simulink model "pos_control2"  (R2016b)
settings: Solver=ode3  StartTime=0.0  StopTime=50  FixedStep=0.0025  RelTol=1e-3
model workspace: external: MATLAB File /home/zhouhua/Clobotics/px4_simulink/px4_motor_order/pos_control_px4_order/para_pos.m (data not in the file)
values from neighbouring files (symbols this model uses):
  Ang_Pos_initial = [x0, y0, z0, phi0, theta0, psi0]    [para_pos.m]
  b = (middle_cruise_speed - c) / a    [get_vel_close.m]    (also in gradual.m = y_low - a * x_low; para_pos.m = 1.38089806e-06)
  compensation_gain = 1    [para_pos.m]
  d = 4.152245751114358e-08    (= 4.15224575111e-08)    [para_pos.m]
  dt = 0.0025    [para_pos.m]
  g = 9.8    [para_pos.m]
  Ix = 0.676603    [para_pos.m]
  Iy = 0.996394    [para_pos.m]
  Iz = 0.640393    [para_pos.m]
  L = 0.6    [para_pos.m]
  m = 10.3551    [para_pos.m]
  omiga1 = 0000    (= 0)    [para_pos.m]
  omiga2 = 0000    (= 0)    [para_pos.m]
  omiga3 = 0000    (= 0)    [para_pos.m]
  omiga4 = 0000    (= 0)    [para_pos.m]
  thrust_rpyt_low = [0,0,0,0,0,0]    [para_pos.m]
  thrust_rpyt_up = [1,1,1,1,1,1]    [para_pos.m]
  X1_PWM_MotorVel = -0.0023    [para_pos.m]
  X2_PWM_MotorVel = 13.6492    [para_pos.m]
  X3_PWM_MotorVel = -1.2185e+4    (= -12185)    [para_pos.m]
undefined symbols (not defined in the file or in its folder): bool_pos, control_mode, def, par, par_input, par_pos, position_setpoint
libraries: simulink x1
(part 2 of 2)

== matlab function pos_control2/position_control/control_auto ==
  data: prev_pos_sp input; next_sp input; curr_pos_sp input; pos input; vel input; att_euler input; vel_sp_prev input; pos_sp_prev input; att_sp_prev_yaw_body input; pos_sp_x output; pos_sp_y output; pos_sp_z output; vel_sp_x output; vel_sp_y output; vel_sp_z output; att_sp_yaw_body output; vel_max_xy output; def parameter; bool_pos parameter; position_setpoint parameter; par_pos parameter; dt parameter
function [pos_sp_x,pos_sp_y,pos_sp_z,vel_sp_x,vel_sp_y,vel_sp_z,att_sp_yaw_body,vel_max_xy] = control_auto(prev_pos_sp,next_sp,curr_pos_sp,pos,vel,att_euler,vel_sp_prev,pos_sp_prev,att_sp_prev_yaw_body,def, bool_pos, position_setpoint,par_pos, dt)
%curr_pos_sp(valid,type,x,y,z,vx,vy,vz,ax,ay,az,yaw,yawspeed,cruising_speed,position_valid,velocity_valid,acceleration_valid,yaw_valid,yawspeed_valid,cruising_valid)
%[1,0,10,10,10,0.1,0.1,0.1,0,0,0,1,0.1,0,1,1,0,1,0,0]
%prev_sp,next_sp [valid,type,x,y,z]
vel_max_xy = par_pos.vel_max_xy;
pos_sp = zeros(3,1);
pos_sp = pos_sp_prev;
vel_sp = zeros(3,1);
vel_sp = vel_sp_prev;
yaw = att_euler(3);
att_sp_yaw_body = att_sp_prev_yaw_body;
% reset position setpoint on AUTO mode activation or if we are not in MC mode */
if ~bool_pos.mode_auto
    bool_pos.mode_auto = 1;
    %set _triplet_lat_lon_finite true once switch to AUTO(e.g. LAND)
    bool_pos.triplet_lat_lon_finite = 1;

end

bool_pos.reset_pos_sp = 1;
bool_pos.reset_alt_sp = 1;

% Always check reset state of altitude and position control flags in auto
if (bool_pos.reset_pos_sp)
   bool_pos.reset_pos_sp = 0;
   pos_sp(1) = pos(1);
   pos_sp(2) = pos(2);
end

if (bool_pos.reset_alt_sp)
    bool_pos.reset_alt_sp = 0;
    pos_sp(3) = pos(3);
end

% init bool and vector
%bool
current_setpoint_valid = 0;
previous_setpoint_valid = 0;
next_setpoint_valid = 0;
triplet_updated = 0;

if (curr_pos_sp(1))

    %math::Vector<3> 
    %curr_pos_sp = _curr_pos_sp;

    %only project setpoints if they are finite, else use current position
     
    %if (PX4_ISFINITE(_pos_sp_triplet.current.lat) &&
       % PX4_ISFINITE(_pos_sp_triplet.current.lon)) {
        % project setpoint to local frame */
        %map_projection_project(&_ref_pos, _pos_sp_triplet.current.lat, _pos_sp_triplet.current.lon,&curr_pos_sp.data[0], &curr_pos_sp.data[1]);

        %_triplet_lat_lon_finite = true;

    %} else { % use current position if NAN -> e.g. land
       % if (_triplet_lat_lon_finite) {
        %    curr_pos_sp.data[0] = _pos(0);
         %   curr_pos_sp.data[1] = _pos(1);
       %     _triplet_lat_lon_finite = false;
        %}
    % only project setpoints if they are finite, else use current position
    % todo ref_alt
    %if (PX4_ISFINITE(_pos_sp_triplet.current.alt)) {
        %curr_pos_sp(5) = -(_pos_sp_triplet.current.alt - _ref_alt);
   % }
    % sanity check */
    if (isreal(curr_pos_sp(3)) && isreal(curr_pos_sp(4)) && isreal(curr_pos_sp(5)))
        current_setpoint_valid = 1;
    end

    % check if triplets have been updated
    % note: we only can look at xy since navigator applies slewrate to z */
    %float  diff;
    %if (_triplet_lat_lon_finite) {
       % diff = matrix::Vector2f((_curr_pos_sp(0) - curr_pos_sp(0)), (_curr_pos_sp(1) - curr_pos_sp(1))).length();
    %} else {
       % diff = fabsf(_curr_pos_sp(2) - curr_pos_sp(2));
    %}
    %if (diff > FLT_EPSILON) {
    %    triplet_updated = true;
    %}
    % we need to update _curr_pos_sp always since navigator applies slew rate on z */
    %_curr_pos_sp = curr_pos_sp;
end

if (prev_pos_sp(1))
    if (isreal(prev_pos_sp(3)) && isreal(prev_pos_sp(4)) && isreal(prev_pos_sp(5)))
        %_prev_pos_sp = prev_sp;
        previous_setpoint_valid = 1;
    end
end

% set previous setpoint to current position if no previous setpoint available */
if (~previous_setpoint_valid && triplet_updated)
    prev_pos_sp(3) = pos(1);
    prev_pos_sp(4) = pos(2);
    prev_pos_sp(5) = pos(3);
    previous_setpoint_valid = 1; % currrently not necessary to set to true since not used*/
end

if (next_sp(1))
    if (isreal(next_sp(3)) && isreal(next_sp(4)) && isreal(next_sp(5)))
        next_setpoint_valid = 1;
    end
end

%change curr_pos_sp, prev_pos_sp, next_sp
%todo
%current_setpoint_valid = 1;

%create new _pos_sp from triplets
if (current_setpoint_valid && curr_pos_sp(2) ~= position_setpoint.SETPOINT_TYPE_IDLE)
    % update yaw setpoint if needed
    if (curr_pos_sp(19) && position_setpoint.SETPOINT_TYPE_FOLLOW_TARGET)
        att_sp_yaw_body = att_sp_prev_yaw_body + curr_pos_sp(13)*dt;
    elseif (curr_pos_sp(18))
        att_sp_yaw_body = curr_pos_sp(12);
    end
    
    yaw_diff = wrap_pi(att_sp_yaw_body - yaw);
    
    % only follow previous-current-line for specific triplet type
    
    if  (curr_pos_sp(2) == position_setpoint.SETPOINT_TYPE_POSITION  ||curr_pos_sp(2) == position_setpoint.SETPOINT_TYPE_LOITER ||curr_pos_sp(2) == position_setpoint.SETPOINT_TYPE_FOLLOW_TARGET)
        %by default use current setpoint as is
        pos_sp = [curr_pos_sp(3);curr_pos_sp(4);curr_pos_sp(5)];
        
        %Z-DIRECTION
        
        % get various distances
        
		total_dist_z = abs(curr_pos_sp(5) - prev_pos_sp(5));
		dist_to_prev_z = abs(pos(3) - prev_pos_sp(5));
		dist_to_current_z = abs(curr_pos_sp(5) - pos(3));
        
        %  if pos_sp has not reached target setpoint (=curr_pos_sp(2)),
		%  then compute setpoint depending on vel_max
        if (total_dist_z >  def.SIGMA_NORM) && (abs(pos_sp(3) - curr_pos_sp(5)) > def.SIGMA_NORM)
            %%% ???
            flying_upward = (curr_pos_sp(5) < pos(3));
            
            % final_vel_z is the max velocity which depends on the distance of total_dist_z
			% with default params.vel_max_up/down
            if flying_upward
                final_vel_z = par_pos.vel_max_up;
            else
                final_vel_z = par_pos.vel_max_down;
            end
            % target threshold defines the distance to _curr_pos_sp(2) at which
			% the vehicle starts to slow down to approach the target smoothly
            target_threshold_z = final_vel_z * 1.5;
            % if the total distance in z is NOT 2x distance of target_threshold, we
			% will need to adjust the final_vel_z
			is_2_target_threshold_z = total_dist_z >= 2.0 * target_threshold_z;
			
            slope = (final_vel_z) / (target_threshold_z); % defines the the acceleration when slowing down */
			min_vel_z = 0.2; % minimum velocity: this is needed since estimation is not perfect
            
            if (~is_2_target_threshold_z)
				% adjust final_vel_z since we are already very close
				% to current and therefore it is not necessary to accelerate
				% up to full speed (=final_vel_z)
				target_threshold_z = total_dist_z * 0.5;
				%get the velocity at target_threshold_z */
				final_vel_z_tmp = slope * (target_threshold_z) + min_vel_z;

				%make sure that final_vel_z is never smaller than 0.5 of the default final_vel_z
				%this is mainly done because the estimation in z is not perfect and therefore
				%it is necessary to have a minimum speed

				final_vel_z = constrain(final_vel_z_tmp, final_vel_z * 0.5, final_vel_z);
            end

			vel_sp_z = final_vel_z;

			%we want to slow down */
            if (dist_to_current_z < target_threshold_z) 
                vel_sp_z = slope * dist_to_current_z + min_vel_z;
            elseif (dist_to_prev_z < target_threshold_z)
				%we want to accelerate */

				acc_z = (vel_sp_z - abs(vel_sp(3))) / dt;
                if flying_upward
                    acc_max = par_pos.acceleration_z_max_up * 0.5;
                else
                    acc_max = par_pos.acceleration_z_max_down * 0.5;
                end
                
                if (acc_z > acc_max)
                    vel_sp_z = par_pos.acceleration_z_max_up * dt + abs(vel_sp(3));
                end

            end

			%if we already close to current, then just take over the velocity that
			%we would have computed if going directly to the current setpoint
            if (vel_sp_z >= (dist_to_current_z * par_pos.pos_p(3)))
				vel_sp_z = dist_to_current_z * par_pos.pos_p(3);
            end

			% make sure vel_sp_z is always positive */
			vel_sp_z = constrain(vel_sp_z, 0.0, final_vel_z);
			% get the sign of vel_sp_z */
            if flying_upward
                vel_sp_z = -vel_sp_z ;
            %else
               % vel_sp_z = vel_sp_z;
            end
			% compute pos_sp(2) */
			pos_sp(3) = pos(3) + vel_sp_z / par_pos.pos_p(3);
        end
        
        
        % XY-DIRECTION


		% line from previous to current and from pos to current */
        vec_prev_to_current = [(curr_pos_sp(3) - prev_pos_sp(3)); (curr_pos_sp(4) - prev_pos_sp(4))];
        vec_pos_to_current = [(curr_pos_sp(3) - pos(1)); (curr_pos_sp(4) - pos(2))];


		% check if we just want to stay at current position */
		pos_sp_diff = [(curr_pos_sp(3) - pos_sp(1)); (curr_pos_sp(4) - pos_sp(2))];
		% bool
        stay_at_current_pos = (curr_pos_sp(2) == position_setpoint.SETPOINT_TYPE_LOITER || ~next_setpoint_valid) && (normest(pos_sp_diff) < def.SIGMA_NORM);

        % only follow line if previous to current has a minimum distance */

		% only follow line if previous to current has a minimum distance */
        if ((normest(vec_prev_to_current)  > par_pos.nav_rad ) && ~stay_at_current_pos) 

			% normalize prev-current line (always > nav_rad) */
			unit_prev_to_current = vec_prev_to_current/normest(vec_prev_to_current);

			% unit vector from current to next */
			unit_current_to_next = [0.0; 0.0];
            
            if (next_setpoint_valid) 
					unit_current_to_next = [(next_sp(3) - pos_sp(1)); (next_sp(4) - pos_sp(2))];
                    if normest(unit_current_to_next) > def.SIGMA_NORM
                        unit_current_to_next = unit_current_to_next/normest(unit_current_to_next);
                    %else
                        %unit_current_to_next;
                    end
            end

			% point on line closest to pos */
			closest_point = [prev_pos_sp(3); prev_pos_sp(4)] + unit_prev_to_current * ([(pos(1) - prev_pos_sp(3)), (pos(2) - prev_pos_sp(4))] * unit_prev_to_current);

			vec_closest_to_current = [(curr_pos_sp(3) - closest_point(1)); (curr_pos_sp(4) - closest_point(2))];

			% compute vector from position-current and previous-position */
			vec_prev_to_pos = [(pos(1) - prev_pos_sp(3)); (pos(2) - prev_pos_sp(4))];

			% current velocity along track */
			vel_sp_along_track_prev = dot([vel_sp(1); vel_sp(2)], unit_prev_to_current);

			% distance to target when brake should occur */
            if (curr_pos_sp(20) == 1 && ~(curr_pos_sp(14) < 0.0))
                %float
                get_cruising_speed_xy = curr_pos_sp(14);
            else
                get_cruising_speed_xy = par_pos.vel_cruise_xy;
            end
            
			target_threshold_xy = 1.5 * get_cruising_speed_xy;

            %bool
			close_to_current = normest(vec_pos_to_current) < target_threshold_xy;
            %bool
			close_to_prev = (normest(vec_prev_to_pos) < target_threshold_xy) && (normest(vec_prev_to_pos) < normest(vec_pos_to_current));

			% indicates if we are at least half the distance from previous to current close to previous */
			%bool
            is_2_target_threshold = normest(vec_prev_to_current) >= 2.0 * target_threshold_xy;

			% check if the current setpoint is behind */
			%bool
            current_behind = dot((vec_pos_to_current * -1.0), unit_prev_to_current) > 0.0;

			% check if the previous is in front */
			%bool 
            previous_in_front = dot(vec_prev_to_pos, unit_prev_to_current) < 0.0;

			% default velocity along line prev-current */
			%float 
            vel_sp_along_track = get_cruising_speed_xy;

		    %compute velocity setpoint along track

			% only go directly to previous setpoint if more than 5m away and previous in front*/
            if (previous_in_front && (normest(vec_prev_to_pos) > 5.0))
                % just use the default velocity along track */
                vel_sp_along_track = normest(vec_prev_to_pos) * par_pos.pos_p(1);
                if (vel_sp_along_track > get_cruising_speed_xy) 
                    vel_sp_along_track = get_cruising_speed_xy;
                end

            elseif (current_behind)
				% go directly to current setpoint */
				vel_sp_along_track = normest(vec_pos_to_current) * par_pos.pos_p(1);
                if (vel_sp_along_track < get_cruising_speed_xy)
                    %vel_sp_along_track = vel_sp_along_track;
                else
                    vel_sp_along_track = get_cruising_speed_xy;
                end

            elseif (close_to_prev)
				% accelerate from previous setpoint towards current setpoint */

				% we are close to previous and current setpoint
				% we first compute the start velocity when close to current septoint and use
				% this velocity as final velocity when transition occurs from acceleration to deceleration.
				% This ensures smooth transition */
				%float 
                final_cruise_speed = get_cruising_speed_xy;
                
                if (~is_2_target_threshold)
                    % set target threshold to half dist pre-current */
                    %float
                    target_threshold_tmp = target_threshold_xy;
                    target_threshold_xy = normest(vec_prev_to_current) * 0.5;
                    if ((target_threshold_xy - par_pos.nav_rad ) < def.SIGMA_NORM)
                        target_threshold_xy = par_pos.nav_rad ;
                    end

					% velocity close to current setpoint with default zero if no next setpoint is available */
					%float 
                    vel_close = 0.0;
					%float 
                    acceptance_radius = 0.0;

					% we want to pass and need to compute the desired velocity close to current setpoint */
                    if (next_setpoint_valid &&  ~(curr_pos_sp(2) == position_setpoint.SETPOINT_TYPE_LOITER))
                        % get velocity close to current that depends on angle between prev-current and current-next line */
                        vel_close = get_vel_close(get_cruising_speed_xy,unit_prev_to_current, unit_current_to_next);
                        acceptance_radius = par_pos.nav_rad;
                    end

					% compute velocity at transition where vehicle switches from acceleration to deceleration */
                    if ((target_threshold_tmp - acceptance_radius) < def.SIGMA_NORM)
                        final_cruise_speed = vel_close;

                    else
                        %float 
                        slope = (get_cruising_speed_xy - vel_close) / (target_threshold_tmp - acceptance_radius);
                        final_cruise_speed = slope  * (target_threshold_xy - acceptance_radius) + vel_close;
                        if final_cruise_speed > vel_close
                            %final_cruise_speed = final_cruise_speed;
                        else
                            final_cruise_speed = vel_close;
                        end
                    end
                end

				% make sure final cruise speed is larger than 0*/
                if final_cruise_speed > def.SIGMA_NORM
                    %final_cruise_speed = final_cruise_speed;
                else
                    final_cruise_speed = def.SIGMA_NORM;
                end
                
				vel_sp_along_track = final_cruise_speed;

				% we want to accelerate not too fast
				% TODO: change the name acceleration_hor_man to something that can
				% be used by auto and manual */
				
                %float 
                acc_track = (final_cruise_speed - vel_sp_along_track_prev) / dt;

				% if yaw offset is large, only accelerate with 0.5m/s^2 */
				
                %float 
                if (abs(yaw_diff) >  par_pos.mis_yaw_error *def.M_PI_F/180)
                    acc = 0.5;
                else
                    acc = par_pos.acceleration_hor;
                end
                
                if (acc_track > acc)
                    vel_sp_along_track = acc * dt + vel_sp_along_track_prev;
                end

				% enforce minimum cruise speed */
				vel_sp_along_track  = constrain(vel_sp_along_track, def.SIGMA_NORM, final_cruise_speed);
                
            elseif (close_to_current)
				% slow down when close to current setpoint */

				% check if altidue is within acceptance radius */
                %bool 
                if dist_to_current_z < par_pos.nav_rad
                    reached_altitude = 1;
                else
                    reached_altitude = 0;
                end
                
                if (reached_altitude && next_setpoint_valid && ~(curr_pos_sp(2) == position_setpoint.SETPOINT_TYPE_LOITER))
                    % since we have a next setpoint use the angle prev-current-next to compute velocity setpoint limit */

					% get velocity close to current that depends on angle between prev-current and current-next line */
                    %float 
                    vel_close = get_vel_close(get_cruising_speed_xy,unit_prev_to_current, unit_current_to_next);

					% compute velocity along line which depends on distance to current setpoint */
                    if (normest(vec_closest_to_current) < par_pos.nav_rad)
						vel_sp_along_track = vel_close;
                    else
                        if (target_threshold_xy - par_pos.nav_rad < def.SIGMA_NORM)
							vel_sp_along_track = vel_close;
                        else
							%float 
                            slope = (get_cruising_speed_xy - vel_close) / (target_threshold_xy - par_pos.nav_rad) ;
							vel_sp_along_track = slope  * (normest(vec_closest_to_current) - par_pos.nav_rad) + vel_close;
                        end
                    end

					% since we want to slow down take over previous velocity setpoint along track if it was lower */
                    if ((vel_sp_along_track_prev < vel_sp_along_track) && (vel_sp_along_track * vel_sp_along_track_prev > 0.0))
							vel_sp_along_track = vel_sp_along_track_prev;
                    end

					% if we are close to target and the previous velocity setpoints was smaller than
					% vel_sp_along_track, then take over the previous one
					% this ensures smoothness since we anyway want to slow down
                    if ((vel_sp_along_track_prev < vel_sp_along_track) && (vel_sp_along_track * vel_sp_along_track_prev > 0.0) && (vel_sp_along_track_prev > vel_close)) 
                        vel_sp_along_track = vel_sp_along_track_prev;
                    end

					% make sure that vel_sp_along track is at least min */
                    if vel_sp_along_track < vel_close
                        vel_sp_along_track = vel_close;
                    end
				else 

					% we want to stop at current setpoint */
					%float 
                    slope = (get_cruising_speed_xy)  / target_threshold_xy;
					vel_sp_along_track =  slope * (normest(vec_closest_to_current));

					% since we want to slow down take over previous velocity setpoint along track if it was lower but ensure its not zero */
                    if ((vel_sp_along_track_prev < vel_sp_along_track) && (vel_sp_along_track * vel_sp_along_track_prev > 0.0) && (vel_sp_along_track_prev > 0.5)) 
                        vel_sp_along_track = vel_sp_along_track_prev;
                    end
                end
            end
            
            % compute velocity orthogonal to prev-current-line to position*/
            %matrix::Vector2f 
            vec_pos_to_closest = closest_point - [pos(1); pos(2)];
            %float 
            vel_sp_orthogonal = normest(vec_pos_to_closest) * par_pos.pos_p(1);

			% compute the cruise speed from velocity along line and orthogonal velocity setpoint */
            %float 
            cruise_sp_mag = sqrt(vel_sp_orthogonal * vel_sp_orthogonal + vel_sp_along_track * vel_sp_along_track);

			% sanity check *
            if ~isreal(cruise_sp_mag)
                cruise_sp_mag = vel_sp_orthogonal;
            end

			% orthogonal velocity setpoint is smaller than cruise speed */
            if (vel_sp_orthogonal < get_cruising_speed_xy && ~current_behind)

                % we need to limit vel_sp_along_track such that cruise speed  is never exceeded but still can keep velocity orthogonal to track */
                if (cruise_sp_mag > get_cruising_speed_xy)
					vel_sp_along_track = sqrt(get_cruising_speed_xy * get_cruising_speed_xy - vel_sp_orthogonal * vel_sp_orthogonal);
                end

				pos_sp(1) = closest_point(1) + unit_prev_to_current(1) * vel_sp_along_track / par_pos.pos_p(1);
				pos_sp(2) = closest_point(2) + unit_prev_to_current(2) * vel_sp_along_track / par_pos.pos_p(2);
            elseif (current_behind)
                % current is behind */
                if (normest(vec_pos_to_current)  > 0.01) 
                    pos_sp(1) = pos(1) + vec_pos_to_current(1) / normest(vec_pos_to_current) * vel_sp_along_track / par_pos.pos_p(1);
                    pos_sp(2) = pos(2) + vec_pos_to_current(2) / normest(vec_pos_to_current) * vel_sp_along_track / par_pos.pos_p(2);

                else
                    pos_sp(1) = curr_pos_sp(3);
                    pos_sp(2) = curr_pos_sp(4);
                end
            else
                % we are more than cruise_speed away from track */
                % if previous is in front just go directly to previous point */
                if (previous_in_front)
                    vec_pos_to_closest(1) = prev_pos_sp(3) - pos(1);
                    vec_pos_to_closest(2) = prev_pos_sp(4) - pos(2);
                end
                
                % make sure that we never exceed maximum cruise speed */
                %float 
                cruise_sp = normest(vec_pos_to_closest) * par_pos.pos_p(1);
                
                if (cruise_sp > get_cruising_speed_xy)
                    cruise_sp = get_cruising_speed_xy;
                end
                
                % sanity check: don't divide by zero */
                if (normest(vec_pos_to_closest) > def.SIGMA_NORM)
                    pos_sp(1) = pos(1) + vec_pos_to_closest(1) / normest(vec_pos_to_closest) * cruise_sp / par_pos.pos_p(1);
                    pos_sp(2) = pos(2) + vec_pos_to_closest(2) / normest(vec_pos_to_closest) * cruise_sp / par_pos.pos_p(2);
                else
                    pos_sp(1) = closest_point(1);
                    pos_sp(2) = closest_point(2);
                end
            end
        end
        %pos_sp = pos_sp;
    elseif (curr_pos_sp(2) == position_setpoint.SETPOINT_TYPE_VELOCITY)
        if (curr_pos_sp(20) == 1 && ~(curr_pos_sp(14) < 0.0))
            %float
            get_cruising_speed_xy = curr_pos_sp(14);
        else
            get_cruising_speed_xy = par_pos.vel_cruise_xy;
        end

        %float 
        vel_xy_mag = sqrt(vel(1) * vel(1) + vel(2) * vel(2));

        if (vel_xy_mag > def.SIGMA_NORM)
            vel_sp(1) = vel(1) / vel_xy_mag * get_cruising_speed_xy;
            vel_sp(2) = vel(2) / vel_xy_mag * get_cruising_speed_xy;

        else
            % TODO: we should go in the direction we are heading
            % if current velocity is zero
            %
            vel_sp(1) = 0.0;
            vel_sp(2) = 0.0;
        end

        bool_pos.run_pos_control = 0;

    else
        % just go to the target point */;
        pos_sp(1) = curr_pos_sp(3);
        pos_sp(2) = curr_pos_sp(4);
        pos_sp(3) = curr_pos_sp(5);
        
        if (curr_pos_sp(20) == 1 && ~(curr_pos_sp(14) < 0.0))
            %float
            get_cruising_speed_xy = curr_pos_sp(14);
        else
            get_cruising_speed_xy = par_pos.vel_cruise_xy;
        end

        % set max velocity to cruise */
        vel_max_xy = get_cruising_speed_xy;
    end
    

    % sanity check */
    if (~(isreal(pos_sp(1)) && isreal(pos_sp(2)) && isreal(pos_sp(3))))

        %warn_rate_limited("Auto: Position setpoint not finite");
        pos_sp(1) = curr_pos_sp(3);
        pos_sp(2) = curr_pos_sp(4);
        pos_sp(3) = curr_pos_sp(5);
    end
    
    % if we're already near the current takeoff setpoint don't reset in case we switch back to posctl.
    % this makes the takeoff finish smoothly.
	% todo
else
    vel_sp = zeros(3,1);
    bool_pos.run_pos_control = 0;
	bool_pos.run_alt_control = 0;
end


pos_sp_x = pos_sp(1);
pos_sp_y = pos_sp(2);
pos_sp_z = pos_sp(3);
vel_sp_x = vel_sp(1);
vel_sp_y = vel_sp(2);
vel_sp_z = vel_sp(3);

== matlab function pos_control2/position_control/control_position ==
  data: vel_sp_prev_x input; vel_sp_prev_y input; vel_sp_prev_z input; pos_sp_prev_x input; pos_sp_prev_y input; pos_sp_prev_z input; pos input; vel input; curr_pos_sp input; att_euler input; vehicle_land_detected input; takeoff_vel_limit input; att_sp_yaw_body input; vel_max_xy input; vel_sp output; pos_sp output; att_sp output; att_sp_3 output; local_pos_sp_acc output; judge_auto_enable output; thrust_int_prev input; State_prev input; input_prev input; thrust_int output; def parameter; bool_pos parameter; par_pos parameter; control_mode parameter; par_input parameter; position_setpoint parameter; State output; input output; thrust_sp output; saturation_xy output; saturation_z output; vel_err output; testbool output; thrust_body_z output; R_z output; R_set_output output; body_z output; dt parameter
function [vel_sp,pos_sp,att_sp,att_sp_3,local_pos_sp_acc,judge_auto_enable,thrust_int,State,input,thrust_sp,saturation_xy,saturation_z,vel_err,testbool,thrust_body_z,R_z,R_set_output,body_z] = control_position(vel_sp_prev_x,vel_sp_prev_y,vel_sp_prev_z, pos_sp_prev_x,pos_sp_prev_y,pos_sp_prev_z, pos, vel, curr_pos_sp, att_euler, vehicle_land_detected, takeoff_vel_limit, att_sp_yaw_body,vel_max_xy, thrust_int_prev,State_prev,input_prev,def, bool_pos, par_pos, control_mode, par_input, position_setpoint,dt)
% run position & altitude controllers, if enabled (otherwise use already computed velocity setpoints) */
% prev_pos_sp(x,y,z,type,yaw_valid,yawspeed_valid,yaw,yawspeed,cruising_speed,cruising_valid,acceleration_valid,ax,ay,az)
%prev_pos_sp(valid,type,x,y,z,vx,vy,vz,ax,ay,az,yaw,yawspeed,cruising_speed,position_valid,velocity_valid,acceleration_valid,yaw_valid,yawspeed_valid,cruising_valid)

% vehicle_land_detected(bool_landed,bool_freeall,bool_ground_contact,bool_maybe_landed,alt_max)
%[0]
%att_sp(roll_body,pitch_body,yaw_body,q1_d,q2_d,q3_d,q4_d,thrust,q_d_valid)
%_takeoff_vel_limit = 0.5
body_z = zeros(3,1);
input = zeros(3,1);
R_set_output = zeros(9,1);
vel_err = zeros(3,1);
thrust_sp = zeros(3,1);
R_z = zeros(3,1);
thrust_body_z = 0;
%bool 
saturation_xy = 0;
%bool 
saturation_z = 0;
testbool = bool_pos.reset_int_xy;

vel_sp_prev = [vel_sp_prev_x,vel_sp_prev_y,vel_sp_prev_z]';
pos_sp_prev = [pos_sp_prev_x,pos_sp_prev_y,pos_sp_prev_z];
pos_sp = pos_sp_prev;
vel_sp = vel_sp_prev;
State = State_prev;

thrust_int = thrust_int_prev;
att_sp = zeros(9,1);
att_sp_3 = zeros(3,1);
att_sp(3) = att_sp_yaw_body;
R = euler_to_dcm(att_euler);
R_setpoint = zeros(3,3);
local_pos_sp_acc = zeros(3,1);
judge_auto_enable = 1;

if (bool_pos.run_pos_control)
    % If for any reason, we get a NaN position setpoint, we better just stay where we are.
    if (isreal(pos_sp(1)) && isreal(pos_sp(2)))
        vel_sp(1) = (pos_sp(1) - pos(1)) * par_pos.pos_p(1);
        vel_sp(2) = (pos_sp(2) - pos(2)) * par_pos.pos_p(2);
    else
        vel_sp(1) = 0.0;
        vel_sp(2) = 0.0;
        %warn_rate_limited("Caught invalid pos_sp in x and y");
    end
end

% in auto the setpoint is already limited by the navigator */

if (~control_mode.flag_control_auto_enabled)
    %limit_altitude();
    
    if (vehicle_land_detected(5) < 0.0)
        judge_auto_enable = 0;
    % there is no altitude limitation present
    %return;
    end

    %float 
    altitude_above_home = -(pos(3) - par_input.home_pos(3));

    if (bool_pos.run_alt_control && (altitude_above_home > vehicle_land_detected(5)))
        % we are above maximum altitude
        pos_sp(3) = -vehicle_land_detected(5) +  par_input.home_pos(3);

    elseif (~bool_pos.run_alt_control && vel_sp(3) <= 0.0)
        % we want to fly upwards: check if vehicle does not exceed altitude

        % time to reach zero velocity
        %float 
        delta_t = -vel(3) / par_pos.acceleration_z_max_down;

        % predict next position based on current position, velocity, max acceleration downwards and time to reach zero velocity
        %float 
        pos_z_next = pos(3) + vel(3) * delta_t + 0.5 * par_pos.acceleration_z_max_down * delta_t *delta_t;

        if (-(pos_z_next - par_input.home_pos(3)) > vehicle_land_detected(5))
            % prevent the vehicle from exceeding maximum altitude by switching back to altitude control with maximum altitude as setpoint
            pos_sp(3) = -vehicle_land_detected(5) + par_input.home_pos(3);
            % test 
            %bool_pos.run_alt_control = 1;
        end
    end
end

if (bool_pos.run_alt_control)
    if (isreal(pos_sp(3)))
        vel_sp(3) = (pos_sp(3) - pos(3)) * par_pos.pos_p(3);

    else
        vel_sp(3) = 0.0;
        %warn_rate_limited("Caught invalid pos_sp in z");
    end
end


if (~control_mode.flag_control_position_enabled)
    %bool_pos.reset_pos_sp = 1;
end

if (~control_mode.flag_control_altitude_enabled)
    %bool_pos.reset_alt_sp = 1;
end

if (~control_mode.flag_control_velocity_enabled)
    %vel_sp_prev(1) = vel(1);
    %vel_sp_prev(2) = vel(2);
    vel_sp(1) = 0.0;
    vel_sp(2) = 0.0;
end

if (~control_mode.flag_control_climb_rate_enabled)
    vel_sp(3) = 0.0;
end

% limit vertical upwards speed in auto takeoff and close to ground */
%float 
altitude_above_home = -pos(3) + par_input.home_pos(3);

if (curr_pos_sp(2) == position_setpoint.SETPOINT_TYPE_TAKEOFF && ~control_mode.flag_control_manual_enabled)
    %float 
    vel_limit = gradual(altitude_above_home, par_pos.slow_land_alt2, par_pos.slow_land_alt1, par_pos.tko_speed, par_pos.vel_max_up);
    vel_sp(3) = max(vel_sp(3), -vel_limit);
end

% limit vertical downwards speed (positive z) close to ground
% for now we use the altitude above home and assume that we want to land at same height as we took off */
%float 
vel_limit = gradual(altitude_above_home, par_pos.slow_land_alt2, par_pos.slow_land_alt1, par_pos.land_speed, par_pos.vel_max_down);

vel_sp(3) = min(vel_sp(3), vel_limit);

% apply slewrate (aka acceleration limit) for smooth flying */

if (~control_mode.flag_control_auto_enabled)
    %todo
    %vel_sp_slewrate(dt);
    %matrix::Vector2f 
    vel_sp_xy = [vel_sp(1), vel_sp(2)]';
	%matrix::Vector2f 
    vel_sp_prev_xy = [vel_sp_prev(1), vel_sp_prev(2)]';
	%matrix::Vector2f 
    vel_xy = [vel(1), vel(2)]';
	%matrix::Vector2f 
    acc_xy = (vel_sp_xy - vel_sp_prev_xy)/ dt;

	% limit total horizontal acceleration */
    if (normest(acc_xy) > par_pos.acceleration_state_dependent_xy)
		vel_sp_xy = par_pos.acceleration_state_dependent_xy * acc_xy/normest(acc_xy) * dt + vel_sp_prev_xy;
		vel_sp(1) = vel_sp_xy(1);
		vel_sp(2) = vel_sp_xy(2);
    end

	% limit vertical acceleration */
	%float 
    acc_z = (vel_sp(3) - vel_sp_prev(3)) / dt;
	%float 
    %max_acc_z;

    if (control_mode.flag_control_manual_enabled)
        if acc_z < 0.0
            max_acc_z = -par_pos.acceleration_state_dependent_z;
        else
            max_acc_z = par_pos.acceleration_state_dependent_z;
        end
    else
        if acc_z < 0.0
            max_acc_z = -par_pos.acceleration_z_max_up;
        else
            max_acc_z = par_pos.acceleration_z_max_up;
        end
    end
    
    if (abs(acc_z) > abs(max_acc_z))
		vel_sp(3) = max_acc_z * dt + vel_sp_prev(3);
    end
end

%vel_sp_prev = vel_sp;

% special velocity setpoint limitation for smooth takeoff (after slewrate!) */
if (bool_pos.in_smooth_takeoff)
    if (takeoff_vel_limit < -vel_sp(3))
        %bool_pos.in_smooth_takeoff = 1;
    else
        %bool_pos.in_smooth_takeoff = 0;
    end
    % ramp vertical velocity limit up to takeoff speed */
    takeoff_vel_limit = takeoff_vel_limit -vel_sp(3) * dt / par_pos.takeoff_ramp_time;
    % limit vertical velocity to the current ramp value */
    vel_sp(3) = max(vel_sp(3), -takeoff_vel_limit);
end

% make sure velocity setpoint is constrained in all directions (xyz) */
%float 
vel_norm_xy = sqrt(vel_sp(1) * vel_sp(1) + vel_sp(2) * vel_sp(2));

if (vel_norm_xy > vel_max_xy) 
    vel_sp(1) = vel_sp(1) * vel_max_xy / vel_norm_xy;
    vel_sp(2) = vel_sp(2) * vel_max_xy / vel_norm_xy;
end

vel_sp(3) = constrain(vel_sp(3), -par_pos.vel_max_up, par_pos.vel_max_down);


if (control_mode.flag_control_climb_rate_enabled || control_mode.flag_control_velocity_enabled || control_mode.flag_control_acceleration_enabled)
    	% reset integrals if needed */
    if (control_mode.flag_control_climb_rate_enabled)
        if (bool_pos.reset_int_z)
            %bool_pos.reset_int_z = 0;
            thrust_int(3) = 0.0;
        end
    else
        %bool_pos.reset_int_z = 1;
    end

    if (control_mode.flag_control_velocity_enabled)
        if (bool_pos.reset_int_xy)
            %bool_pos.reset_int_xy = 0;
            thrust_int(1) = 0.0;
            thrust_int(2) = 0.0;
        end
    else
        %bool_pos.reset_int_xy = 1;
    end

    % if any of the velocity setpoint is bogus, it's probably safest to command no velocity at all. */
    for i = 1:3
        if (~isreal(vel_sp(i)))
            vel_sp(i) = 0.0;
        end
    end

    % velocity error */
    vel_err = vel_sp - vel;

    % thrust vector in NED frame */
    thrust_sp = zeros(3,1);
    
    %if (_control_mode.flag_control_acceleration_enabled && _pos_sp_triplet.current.acceleration_valid) {
    %thrust_sp = math::Vector<3>(_pos_sp_triplet.current.a_x, _pos_sp_triplet.current.a_y, _pos_sp_triplet.current.a_z);
    if (control_mode.flag_control_acceleration_enabled && curr_pos_sp(17))
        thrust_sp = [curr_pos_sp(9), curr_pos_sp(10), curr_pos_sp(11)]';
    else
        %todo
        %float 
        %float 
        input = -[vel(1),vel(2),vel(3)]';
        input2 = (input-input_prev)/dt;
        
        b = 2 * def.M_PI_F * 5 * dt;
        %float 
        a = b / (1 + b);
        %set
        State = (a * input2 + (1 - a)*State_prev);
        
        vel_err_d = State;
        thrust_sp = vel_err.*(par_pos.vel_p) + vel_err_d.*(par_pos.vel_d) + thrust_int - [0, 0, par_pos.thr_hover]';
    end

    if (~control_mode.flag_control_velocity_enabled && ~control_mode.flag_control_acceleration_enabled)
        thrust_sp(1) = 0.0;
        thrust_sp(2) = 0.0;
    end
    
    %bool
    in_auto_takeoff =  (curr_pos_sp(2) == position_setpoint.SETPOINT_TYPE_TAKEOFF) || control_mode.flag_control_offboard_enabled;
    %bool
    %todo has no maunal input
    has_manual_control_present = control_mode.flag_control_manual_enabled; % && manual.timestamp > 0;
	% Manual takeoff is triggered if the throttle stick is above 65%.
	manual_wants_takeoff = has_manual_control_present; % && manual.z > 0.65;
    
    if (~in_auto_takeoff && ~manual_wants_takeoff)
        if (vehicle_land_detected(3))
            % if still or already on ground command zero xy thrust_sp in body
            % frame to consider uneven ground */

            % thrust setpoint in body frame*/
            %math::Vector<3> 
            thrust_sp_body = R' * thrust_sp;

            % we dont want to make any correction in body x and y*/
            thrust_sp_body(1) = 0.0;
            thrust_sp_body(2) = 0.0;

            % make sure z component of thrust_sp_body is larger than 0 (positive thrust is downward) */
            if thrust_sp(3) > 0.0
                thrust_sp_body(3) = thrust_sp(3);
            else
                thrust_sp_body(3) = 0;
            end

            % convert back to local frame (NED) */
            thrust_sp = R * thrust_sp_body;
        end

        if (vehicle_land_detected(4))
            % we set thrust to zero
            % this will help to decide if we are actually landed or not
            
            thrust_sp = zeros(3,1);
        end
    end

    if (~control_mode.flag_control_climb_rate_enabled && ~control_mode.flag_control_acceleration_enabled)
        thrust_sp(3) = 0.0;
    end

    % limit thrust vector and check for saturation */
    %bool 
    saturation_xy = 0;
    %bool 
    saturation_z = 0;

    % limit min lift */
    %float 
    thr_min = par_pos.thr_min;

    if (~control_mode.flag_control_velocity_enabled && thr_min < 0.0)
        % don't allow downside thrust direction in manual attitude mode */
        thr_min = 0.0;
    end

    %float 
    tilt_max = par_pos.tilt_max_air;
    %float 
    thr_max = par_pos.thr_max;

    % We can only run the control if we're already in-air, have a takeoff setpoint,
    % or if we're in offboard control.
    % Otherwise, we should just bail out
    if (vehicle_land_detected(1) && ~in_auto_takeoff && ~manual_wants_takeoff)
        % Keep throttle low while still on ground.
        thr_max = 0.0;

    elseif (~control_mode.flag_control_manual_enabled && curr_pos_sp(2) == position_setpoint.SETPOINT_TYPE_LAND)
        % adjust limits for landing mode */
        % limit max tilt and min lift when landing */
        tilt_max = par_pos.tilt_max_land;
    end

    % limit min lift */
    if (-thrust_sp(3) < thr_min)
        thrust_sp(3) = -thr_min;
        % Don't freeze altitude integral if it wants to throttle up */
        if vel_err(3) > 0.0
            saturation_z = 1;
        end
    end

    if (control_mode.flag_control_velocity_enabled || control_mode.flag_control_acceleration_enabled)

        % limit max tilt */
        if (thr_min >= 0.0 && tilt_max < def.M_PI_F / 2 - 0.05)
            % absolute horizontal thrust */
            %float 
            thrust_sp_xy_len = normest([thrust_sp(1), thrust_sp(2)]);

            if (thrust_sp_xy_len > 0.01)
                % max horizontal thrust for given vertical thrust*/
                %float 
                thrust_xy_max = -thrust_sp(3) * tan(tilt_max);

                if (thrust_sp_xy_len > thrust_xy_max)
                    %float 
                    k = thrust_xy_max / thrust_sp_xy_len;
                    thrust_sp(1) = thrust_sp(1)*k;
                    thrust_sp(2) = thrust_sp(2)*k;
                    % Don't freeze x,y integrals if they both want to throttle down */
                    if (vel_err(1) * vel_sp(1) < 0.0) && (vel_err(2) * vel_sp(2) < 0.0)
                    else
                        saturation_xy = 1;
                    end
                end
            end
        end
    end


    if (control_mode.flag_control_climb_rate_enabled && ~control_mode.flag_control_velocity_enabled)
        % thrust compensation when vertical velocity but not horizontal velocity is controlled */
        %float 
        %att_comp;

        %const float 
        tilt_cos_max = 0.7;

        if (R(3, 3) > tilt_cos_max)
            att_comp = 1.0 / R(3, 3);

        elseif (R(3, 3) > 0.0)
            att_comp = ((1.0 / tilt_cos_max - 1.0) / tilt_cos_max) * R(3, 3) + 1.0;
            saturation_z = 1;

        else
            att_comp = 1.0;
            saturation_z = 1;
        end

        thrust_sp(3) =thrust_sp(3)* att_comp;
    end
    

    % Calculate desired total thrust amount in body z direction. */
    % To compensate for excess thrust during attitude tracking errors we
    % project the desired thrust force vector F onto the real vehicle's thrust axis in NED:
    % body thrust axis [0,0,-1]' rotated by R is: R*[0,0,-1]' = -R_z */
    %matrix::Vector3f 
    R_z=[R(1, 3), R(2, 3), R(3, 3)]';
    %matrix::Vector3f 
    F = thrust_sp;
    %float 
    thrust_body_z = dot(F, -R_z); % recalculate because it might have changed */

    % limit max thrust */
    if (abs(thrust_body_z) > thr_max)
        if (thrust_sp(3) < 0.0)
            if (-thrust_sp(3) > thr_max)
                % thrust Z component is too large, limit it */
                thrust_sp(1) = 0.0;
                thrust_sp(2) = 0.0;
                thrust_sp(3) = -thr_max;
                saturation_xy = 1;
                % Don't freeze altitude integral if it wants to throttle down */
                if vel_err(3) < 0.0
                    saturation_z = 1;
                end
            else
                % preserve thrust Z component and lower XY, keeping altitude is more important than position */
                %float 
                thrust_xy_max = sqrt(thr_max * thr_max - thrust_sp(3) * thrust_sp(3));
                %float 
                thrust_xy_abs = normest([thrust_sp(1), thrust_sp(2)]);
                %float 
                k = thrust_xy_max / thrust_xy_abs;
                thrust_sp(1) = thrust_sp(1)*k;
                thrust_sp(2) = thrust_sp(2)*k;
                % Don't freeze x,y integrals if they both want to throttle down */
                if (vel_err(1) * vel_sp(1) < 0.0) && (vel_err(2) * vel_sp(2) < 0.0)
                else
                    saturation_xy = 1;
                end
            end
        else
            % Z component is positive, going down (Z is positive down in NED), simply limit thrust vector */
            %float 
            k = thr_max / abs(thrust_body_z);
            thrust_sp = thrust_sp*k;
            saturation_xy = 1;
            saturation_z = 1;
        end
        thrust_body_z = thr_max;
    end

    % if any of the thrust setpoint is bogus, send out a warning */
    %if (~PX4_ISFINITE(thrust_sp(0)) || ~PX4_ISFINITE(thrust_sp(1)) || ~PX4_ISFINITE(thrust_sp(2)))
        %warn_rate_limited("Thrust setpoint not finite");
    % end

    %_att_sp.thrust
    att_sp(8) = max(thrust_body_z, thr_min);

    % update integrals */
    if (control_mode.flag_control_velocity_enabled && ~saturation_xy)
        thrust_int(1) = thrust_int(1) + vel_err(1) * par_pos.vel_i(1) * dt;
        thrust_int(2) = thrust_int(2) + vel_err(2) * par_pos.vel_i(2) * dt;
    end

    if (control_mode.flag_control_climb_rate_enabled && ~saturation_z)
        thrust_int(3) = thrust_int(3) + vel_err(3) * par_pos.vel_i(3) * dt;
    end

    % calculate attitude setpoint from thrust vector */
    if (control_mode.flag_control_velocity_enabled || control_mode.flag_control_acceleration_enabled)
        % desired body_z axis = -normalize(thrust_vector) */
        %math::Vector<3> 
        body_x = zeros(3,1);
        %math::Vector<3> 
        body_y = zeros(3,1);
        %math::Vector<3> 
        body_z = zeros(3,1);

        if (normest(thrust_sp) > def.SIGMA_NORM)
            body_z = -thrust_sp/normest(thrust_sp);

        else
            % no thrust, set Z axis to safe value */
            body_z = zeros(3,1);
            body_z(3) = 1.0;
        end

        % vector of desired yaw direction in XY plane, rotated by PI/2 */
        %math::Vector<3> 
        y_C = [-sin(att_sp(3)), cos(att_sp(3)), 0.0]';

        if (abs(body_z(3)) > def.SIGMA_SINGLE_OP)
            % desired body_x axis, orthogonal to body_z */
            body_x = cross(y_C, body_z);

            % keep nose to front while inverted upside down */
            if (body_z(3) < 0.0)
                body_x = -body_x;
            end

            body_x = body_x/normest(body_x);

        else
            % desired thrust is in XY plane, set X downside to construct correct matrix,
            % but yaw component will not be used actually */
            body_x = zeros(3,1);
            body_x(3) = 1.0;
        end

        % desired body_y axis */
        body_y = cross(body_z, body_x);

        % fill rotation matrix */
        for i = 1:3
            R_setpoint(i, 1) = body_x(i);
            R_setpoint(i, 2) = body_y(i);
            R_setpoint(i, 3) = body_z(i);
        end
        
        R_set_output(1) = R_setpoint(1, 1);
        R_set_output(2) = R_setpoint(1, 2);
        R_set_output(3) = R_setpoint(1, 3);
        R_set_output(4) = R_setpoint(2, 1);
        R_set_output(5) = R_setpoint(2, 2);
        R_set_output(6) = R_setpoint(2, 3);
        R_set_output(7) = R_setpoint(3, 1);
        R_set_output(8) = R_setpoint(3, 2);
        R_set_output(9) = R_setpoint(3, 3);
        % copy quaternion setpoint to attitude setpoint topic */
        %matrix::Quatf 
        q_sp = dcm_to_q(R_setpoint);
        att_sp(4) = q_sp(1);
        att_sp(5) = q_sp(2);
        att_sp(6) = q_sp(3);
        att_sp(7) = q_sp(4);
        att_sp(9) = 1;

        % calculate euler angles, for logging only, must not be used for control */
        %matrix::Eulerf 
        euler = dcm_to_euler(R_setpoint);
        att_sp(1) = euler(1);
        att_sp(2) = euler(2);
        % yaw already used to construct rot matrix, but actual rotation matrix can have different yaw near singularity */

    elseif (~control_mode.flag_control_manual_enabled)
        % autonomous altitude control without position control (failsafe landing),
        % force level attitude, don't change yaw */
        R_setpoint = euler_to_dcm([0.0, 0.0, att_sp(3)]);

        % copy quaternion setpoint to attitude setpoint topic */
        %matrix::Quatf 
        q_sp = q_to_dcm(R_setpoint);
        att_sp(4) = q_sp(1);
        att_sp(5) = q_sp(2);
        att_sp(6) = q_sp(3);
        att_sp(7) = q_sp(4);
        
        att_sp(9) = 1;

        att_sp(1) = 0.0;
        att_sp(2) = 0.0;
    end

    % save thrust setpoint for logging */
    
    local_pos_sp_acc(1) = thrust_sp(1) * def.CONSTANTS_ONE_G;
    local_pos_sp_acc(2)= thrust_sp(2) * def.CONSTANTS_ONE_G;
    local_pos_sp_acc(3) = thrust_sp(3) * def.CONSTANTS_ONE_G;

    %_att_sp.timestamp = hrt_absolute_time();

else
    %bool_pos.reset_int_z = 1;
end

att_sp_3(1) = att_sp(1);
att_sp_3(2) = att_sp(2);
att_sp_3(3) = att_sp(3);

== matlab function pos_control2/model1/ Quadrotor System/Acceleration of X/MATLAB Function ==
  data: Angle input; ddx output; Lift input; m input
function ddx = fcn(Angle, Lift, m)
phi = Angle(1); theta = Angle(2); psi = Angle(3);
ddx = Lift / m *(cos(phi) * sin(theta) * cos(psi) + sin(phi) * sin(psi));

== matlab function pos_control2/model1/ Quadrotor System/Acceleration of Y/MATLAB Function ==
  data: Angle input; ddy output; List input; m input
function ddy = fcn(Angle, List, m)
phi = Angle(1); theta = Angle(2); psi = Angle(3);
ddy = List / m * (cos(phi) * sin(theta) * sin(psi) - sin(phi)*cos(psi));

== matlab function pos_control2/model1/ Quadrotor System/Acceleration of Z/MATLAB Function ==
  data: Angle input; ddz output; List input; m input; g input
function ddz = fcn(Angle, List, m,g)
phi = Angle(1); theta = Angle(2); psi = Angle(3);
ddz = List * ((cos(theta) * cos(phi)) ) / m - g;

== matlab function pos_control2/model1/ Quadrotor System/Acceleration of phi/MATLAB Function ==
  data: Motion_phi input; dd_phi output; Ix input; Iy input; Iz input; Ang_rate input
function dd_phi = fcn(Motion_phi, Ix, Iy, Iz, Ang_rate)
D_theta = Ang_rate(2); D_psi = Ang_rate(3);
dd_phi = D_theta * D_psi * (Iy-Iz) / Ix + Motion_phi / Ix;

== matlab function pos_control2/model1/ Quadrotor System/Acceleration of theta/MATLAB Function ==
  data: Motion_theta input; dd_theta output; Ix input; Iy input; Iz input; Ang_rate input
function dd_theta = fcn(Motion_theta, Ix, Iy, Iz, Ang_rate)
D_phi = Ang_rate(1); D_psi = Ang_rate(3);
dd_theta = D_phi * D_psi * (Iz - Ix) / Iy + Motion_theta / Iy;
